simulink model "Blocks461_S20"  (R2017b)
settings: Solver=ode45  StartTime=0.  StopTime=20  MaxStep=0.01  RelTol=1e-6  AbsTol=1e-6  EnableMultiTasking=on
settings Model: ExtModeTrigMode=oneshot  ExtModeArmWhenConnect=off  Creator=LEVIENKL  LastModifiedBy=carlislt
settings DataIOCC: SaveFormat=Array  SignalLoggingSaveFormat=ModelDataLogs  SaveOutput=off  SaveTime=off  SignalLoggingName=sigsOut
settings OptimizationCC: BlockReduction=off  BooleanDataType=off  ExpressionDepthLimit=2147483647  InitFltsAndDblsToZero=on  LifeSpan=inf
settings DebuggingCC: SaveWithParameterizedLinksMsg=none  UnderspecifiedInitializationDetection=Classic  MergeDetectMultiDrivingBlocksExec=none  SignalResolutionControl=TryResolveAllWithWarning  MultiTaskDSMMsg=warning  MultiTaskCondExecSysMsg=none  FcnCallInpInsideContextMsg=warning  AllowSymbolicDim=off  StateNameClashWarn=warning  SFUnexpectedBacktrackingDiag=warning  SFNoUnconditionalDefaultTransitionDiag=warning  SFExecutionAtInitializationDiag=none
settings HardwareCC: ProdBitPerPointer=32  ProdBitPerSizeT=32  ProdBitPerPtrDiffT=32  ProdLargestAtomicFloat=None  ProdIntDivRoundTo=Undefined  ProdEndianess=Unspecified  ProdWordSize=32  ProdHWDeviceType=32-bit Generic  TargetUnknown=on
settings ModelReferenceCC: PropagateSignalLabelsOutOfModel=off
settings CodeAppCC: StateflowObjectComments=on
settings GRTTargetCC: TargetFcnLib=ansi_tfl_tmw.mat  TargetLangStandard=C89/C90 (ANSI)  GeneratePreprocessorConditionals=Disable all  CombineOutputUpdateFcns=off  GRTInterface=on
settings ConfigComp: CovMetricSettings=dw  CovHtmlReporting=on  CovSaveCumulativeToWorkspaceVar=on  CovSaveSingleToWorkspaceVar=on  CovExternalEMLEnable=off  CovSFcnEnable=off

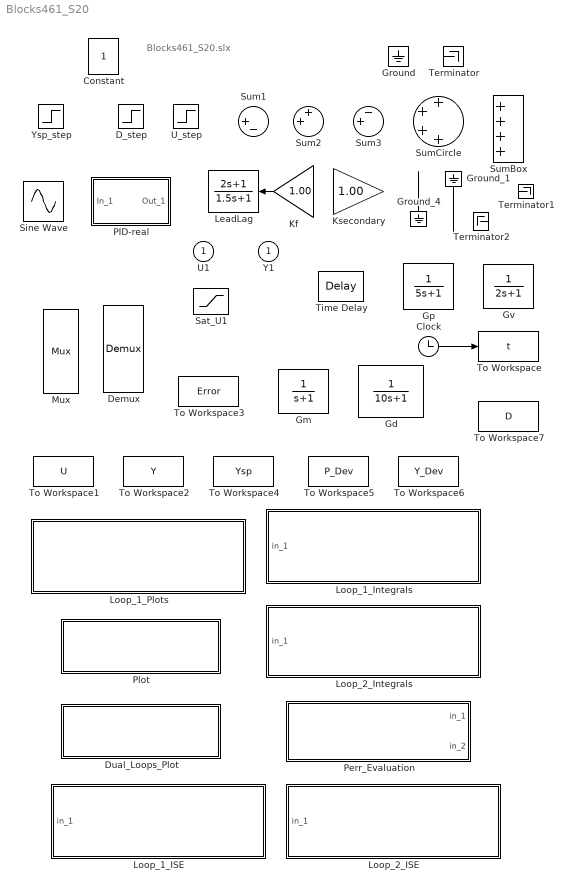
== system Blocks461_S20 ==
  note: Blocks461_S20.slx
  U1 : Inport
  Clock : Clock
  Constant : Constant
  D_step : Step  Time=0  After=0  SampleTime=0
      settings: AttributesFormatString=%<Before> to %<After>\nat %<Time>
  Demux : Demux  Outputs=2
  Dual_Loops_Plot : Subsystem  mask(Daul Y,P Plots 2 Loops){}
      settings: OpenFcn=DualYP
      mask Help: This block two loops Y and P.
      mask Display: disp('After Simulation:\n Double Click for Plots\n (uses DualYP.m)')
  Gd : TransferFcn  Denominator=[10 1]
  Gm : TransferFcn  Denominator=[1 1]
  "Gp " : TransferFcn  Denominator=[5 1]
  Ground : Ground
  Ground_1 : Ground
  Ground_4 : Ground
  Gv : TransferFcn  Denominator=[2 1]
  Kf : Gain  Gain=1.00  SaturateOnIntegerOverflow=on  OutDataTypeStr=Inherit: Same as input  ParamDataTypeStr=Inherit: Same as input
  Ksecondary : Gain  Gain=1.00  SaturateOnIntegerOverflow=on  OutDataTypeStr=Inherit: Same as input  ParamDataTypeStr=Inherit: Same as input
  LeadLag : TransferFcn  Numerator=[2, 1]  Denominator=[1.5, 1]
  Loop_1_ISE : Subsystem  mask(Integral Squarred Evaluation - Loop 1){}
      settings: OpenFcn=ISE1
      mask Help: This block calculates and plots loop #1 ISE.
      mask Display: disp('After Loop 1 Simulation:\n Double Click for ISE evaluation\n (uses ISE1.p)')
  Loop_1_Integrals : Subsystem  mask(Integral Error (3) Evaluations){}
      settings: OpenFcn=I3errs1
      mask Help: This block calculates loop #1 IAE, ISE and ITAE.
      mask Display: disp('After Loop 1 Simulation:\n Double Click for IAE, ISE & ITAE\n (uses I3errs1.p)')
  Loop_1_Plots : Subsystem  mask(Y,U,E Plots - Loop 1){}
      settings: OpenFcn=YPEplots
      mask Help: This block loop #1 Y,U,Error in 3x1 Figure Window.
      mask Display: disp('After Loop 1 Simulation:\n Double Click for Y, P, Error Plots\n (uses YPEplots.p)')
  Loop_2_ISE : Subsystem  mask(Integral Squarred Evaluation - Loop 2){}
      settings: OpenFcn=ISE2
      mask Help: This block calculates and plots loop #2 ISE.
      mask Display: disp('After Loop 2 Simulation:\n Double Click for ISE evaluation\n (uses ISE2.p)')
  Loop_2_Integrals : Subsystem  mask(3 Error evaluations){}
      settings: OpenFcn=I3errs2
      mask Help: This block calculates the IAE, the ISE and the ITAE.
      mask Display: disp('After Loop 2 Simulation:\n Double Click for IAE, ISE & ITAE\n (uses I3errs2.p)')
  Mux : Mux  Inputs=2
  PID-real : Subsystem  mask(PID(with alpha) Controller for ChE 461){Kc=1.00, tauIi=0, tauD=0, alpha=0.05}
      mask prompts: Kc "Controller gain:"; tauIi "Inv of Integral time constant (careful - this is I action ! ) :"; tauD "Derivative time constant:"; alpha "Alpha value (small)::"
      mask help:
      | Enter expressions for controller gain,
      | inverse of integral time constant
      | and derivative time constant and alpha.
      settings: AttributesFormatString=Kc = %<Kc>\n1/TauI = %<tauIi>\nTauD = %<tauD>
      mask Help: This block implements a PID controller where parameters are entered for the Controller Gain, inverse of Integral time constant and Derivative time constant.  Alpha here is equal to 0.01.   Unmask this block to see how it works. The derivative term is implemented using a true derivative block.
      mask Display: disp('PIDalpha')
  Perr_Evaluation : Subsystem  mask(Error evaluation){}
      settings: OpenFcn=Perror
      mask Help: This block calculates the average of the sum of ITAE and ISE for both outputs.
      mask Display: disp('After Project Simulation:\n Double Click for Project Error\n (uses Perror.p)')
  Plot : Subsystem  mask(Y,U,E Plots - Loop 1){}
      settings: OpenFcn=MyPlot
      mask Help: This block loop #1 Y,U,Error in 3x1 Figure Window.
      mask Display: disp('After Simulation:\n Double Click for Plots\n (uses MyPlot.m)')
  Sat_U1 : Saturate  UpperLimit=50  LowerLimit=-50  ZeroCross=off
      settings: AttributesFormatString=%<UpperLimit>\n%<LowerLimit>
  Sine Wave : Sin  SampleTime=0
      settings: AttributesFormatString=|
      | Amp = %<Amplitude>
      | Freq = %<Frequency> rad/t
  Sum1 : Sum  Inputs=|+-  SaturateOnIntegerOverflow=on  InputSameDT=on  OutDataTypeStr=Inherit: Same as first input
  Sum2 : Sum  Inputs=++|  SaturateOnIntegerOverflow=on  InputSameDT=on  OutDataTypeStr=Inherit: Same as first input
  Sum3 : Sum  Inputs=-+|  SaturateOnIntegerOverflow=on  InputSameDT=on  OutDataTypeStr=Inherit: Same as first input
  SumBox : Sum  Inputs=++++
  SumCircle : Sum  Inputs=++++
  Terminator : Terminator
  Terminator1 : Terminator
  Terminator2 : Terminator
  Time Delay : TransportDelay  DelayTime=0.5
      settings: AttributesFormatString=Delay=%<DelayTime>
  To Workspace : ToWorkspace  VariableName=t  SampleTime=-1
  To Workspace1 : ToWorkspace  VariableName=U  SampleTime=-1
  To Workspace2 : ToWorkspace  VariableName=Y  SampleTime=-1
  To Workspace3 : ToWorkspace  VariableName=Error  SampleTime=-1
  To Workspace4 : ToWorkspace  VariableName=Ysp  SampleTime=-1
  To Workspace5 : ToWorkspace  VariableName=P_Dev  SampleTime=-1
  To Workspace6 : ToWorkspace  VariableName=Y_Dev  SampleTime=-1
  To Workspace7 : ToWorkspace  VariableName=D  SampleTime=-1
  U_step : Step  Time=0  After=0  SampleTime=0
      settings: AttributesFormatString=%<Before> to %<After>\nat %<Time>
  Ysp_step : Step  Time=0  After=0  SampleTime=0
      settings: AttributesFormatString=%<Before> to %<After>\nat %<Time>
  Y1 : Outport
  wires:
  Ground_4/1 -> ?
  Ground_1/1 -> ?
  ? -> Terminator1/1
  ? -> Terminator2/1
  Clock/1 -> To Workspace/1
  Kf/1 -> LeadLag/1

== system Blocks461_S20/Dual_Loops_Plot ==

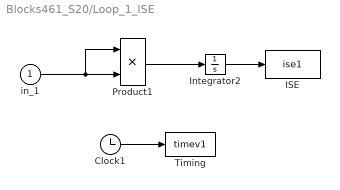
== system Blocks461_S20/Loop_1_ISE ==
  in_1 : Inport
  Clock1 : Clock
  ISE : ToWorkspace  VariableName=ise1
      settings: MaxDataPoints=20000
  Integrator2 : Integrator
  Product1 : Product  SaturateOnIntegerOverflow=on  RndMeth=Zero  InputSameDT=on  OutDataTypeStr=Inherit: Same as first input
  Timing : ToWorkspace  VariableName=timev1
      settings: MaxDataPoints=20000
  wires:
  Product1/1 -> Integrator2/1
  Clock1/1 -> Timing/1
  Integrator2/1 -> ISE/1
  in_1/1 -> Product1/1, Product1/2

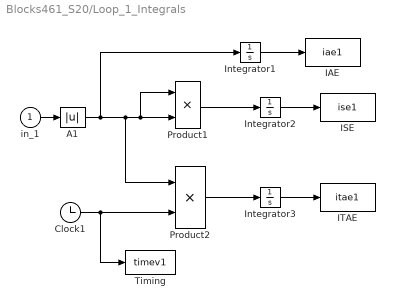
== system Blocks461_S20/Loop_1_Integrals ==
  in_1 : Inport
  A1 : Abs  ZeroCross=off  SaturateOnIntegerOverflow=on
  Clock1 : Clock
  IAE : ToWorkspace  VariableName=iae1
      settings: MaxDataPoints=20000
  ISE : ToWorkspace  VariableName=ise1
      settings: MaxDataPoints=20000
  ITAE : ToWorkspace  VariableName=itae1
      settings: MaxDataPoints=20000
  Integrator1 : Integrator
  Integrator2 : Integrator
  Integrator3 : Integrator
  Product1 : Product  SaturateOnIntegerOverflow=on  RndMeth=Zero  InputSameDT=on  OutDataTypeStr=Inherit: Same as first input
  Product2 : Product  SaturateOnIntegerOverflow=on  RndMeth=Zero  InputSameDT=on  OutDataTypeStr=Inherit: Same as first input
  Timing : ToWorkspace  VariableName=timev1
      settings: MaxDataPoints=20000
  wires:
  Integrator1/1 -> IAE/1
  Product1/1 -> Integrator2/1
  Clock1/1 -> Timing/1, Product2/2
  Integrator3/1 -> ITAE/1
  Integrator2/1 -> ISE/1
  Product2/1 -> Integrator3/1
  A1/1 -> Integrator1/1, Product2/1, Product1/1, Product1/2
  in_1/1 -> A1/1

== system Blocks461_S20/Loop_1_Plots ==

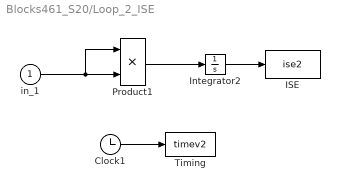
== system Blocks461_S20/Loop_2_ISE ==
  in_1 : Inport
  Clock1 : Clock
  ISE : ToWorkspace  VariableName=ise2
      settings: MaxDataPoints=20000
  Integrator2 : Integrator
  Product1 : Product  SaturateOnIntegerOverflow=on  RndMeth=Zero  InputSameDT=on  OutDataTypeStr=Inherit: Same as first input
  Timing : ToWorkspace  VariableName=timev2
      settings: MaxDataPoints=20000
  wires:
  Product1/1 -> Integrator2/1
  Clock1/1 -> Timing/1
  Integrator2/1 -> ISE/1
  in_1/1 -> Product1/1, Product1/2

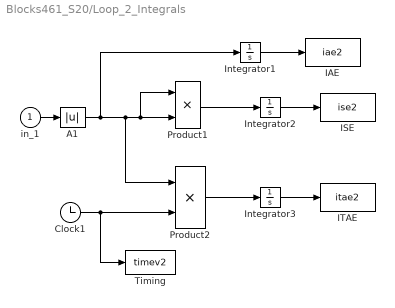
== system Blocks461_S20/Loop_2_Integrals ==
  in_1 : Inport
  A1 : Abs  ZeroCross=off  SaturateOnIntegerOverflow=on
  Clock1 : Clock
  IAE : ToWorkspace  VariableName=iae2
      settings: MaxDataPoints=20000
  ISE : ToWorkspace  VariableName=ise2
      settings: MaxDataPoints=20000
  ITAE : ToWorkspace  VariableName=itae2
      settings: MaxDataPoints=20000
  Integrator1 : Integrator
  Integrator2 : Integrator
  Integrator3 : Integrator
  Product1 : Product  SaturateOnIntegerOverflow=on  RndMeth=Zero  InputSameDT=on  OutDataTypeStr=Inherit: Same as first input
  Product2 : Product  SaturateOnIntegerOverflow=on  RndMeth=Zero  InputSameDT=on  OutDataTypeStr=Inherit: Same as first input
  Timing : ToWorkspace  VariableName=timev2
      settings: MaxDataPoints=20000
  wires:
  Integrator1/1 -> IAE/1
  Product1/1 -> Integrator2/1
  Clock1/1 -> Timing/1, Product2/2
  Integrator3/1 -> ITAE/1
  Integrator2/1 -> ISE/1
  Product2/1 -> Integrator3/1
  A1/1 -> Integrator1/1, Product2/1, Product1/1, Product1/2
  in_1/1 -> A1/1

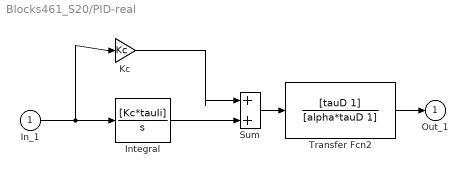
== system Blocks461_S20/PID-real ==
  In_1 : Inport
  Integral : TransferFcn  Numerator=[Kc*tauIi]  Denominator=[1 0]
  Kc : Gain  Gain=Kc  SaturateOnIntegerOverflow=on  OutDataTypeStr=Inherit: Same as input  ParamDataTypeStr=Inherit: Same as input
  Sum : Sum  SaturateOnIntegerOverflow=on  InputSameDT=on  OutDataTypeStr=Inherit: Same as first input
  Transfer Fcn2 : TransferFcn  Numerator=[tauD 1]  Denominator=[alpha*tauD 1]
  Out_1 : Outport
  wires:
  Kc/1 -> Sum/1
  Integral/1 -> Sum/2
  In_1/1 -> Kc/1, Integral/1
  Sum/1 -> Transfer Fcn2/1
  Transfer Fcn2/1 -> Out_1/1

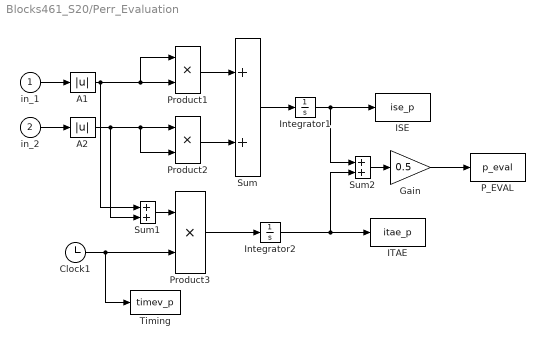
== system Blocks461_S20/Perr_Evaluation ==
  in_1 : Inport
  in_2 : Inport  Port=2
  A1 : Abs  ZeroCross=off  SaturateOnIntegerOverflow=on
  A2 : Abs  ZeroCross=off  SaturateOnIntegerOverflow=on
  Clock1 : Clock
  Gain : Gain  Gain=0.5  SaturateOnIntegerOverflow=on  OutDataTypeStr=Inherit: Same as input  ParamDataTypeStr=Inherit: Same as input
  ISE : ToWorkspace  VariableName=ise_p
      settings: MaxDataPoints=20000
  ITAE : ToWorkspace  VariableName=itae_p
      settings: MaxDataPoints=20000
  Integrator1 : Integrator
  Integrator2 : Integrator
  P_EVAL : ToWorkspace  VariableName=p_eval
      settings: MaxDataPoints=20000
  Product1 : Product  SaturateOnIntegerOverflow=on  RndMeth=Zero  InputSameDT=on  OutDataTypeStr=Inherit: Same as first input
  Product2 : Product  SaturateOnIntegerOverflow=on  RndMeth=Zero  InputSameDT=on  OutDataTypeStr=Inherit: Same as first input
  Product3 : Product  SaturateOnIntegerOverflow=on  RndMeth=Zero  InputSameDT=on  OutDataTypeStr=Inherit: Same as first input
  Sum : Sum  SaturateOnIntegerOverflow=on  InputSameDT=on  OutDataTypeStr=Inherit: Same as first input
  Sum1 : Sum  SaturateOnIntegerOverflow=on  InputSameDT=on  OutDataTypeStr=Inherit: Same as first input
  Sum2 : Sum  SaturateOnIntegerOverflow=on  InputSameDT=on  OutDataTypeStr=Inherit: Same as first input
  Timing : ToWorkspace  VariableName=timev_p
      settings: MaxDataPoints=20000
  wires:
  in_2/1 -> A2/1
  in_1/1 -> A1/1
  Product1/1 -> Sum/1
  Product2/1 -> Sum/2
  Sum/1 -> Integrator1/1
  Sum1/1 -> Product3/1
  A1/1 -> Product1/1, Product1/2, Sum1/1
  A2/1 -> Product2/2, Product2/1, Sum1/2
  Product3/1 -> Integrator2/1
  Integrator1/1 -> Sum2/1, ISE/1
  Integrator2/1 -> Sum2/2, ITAE/1
  Sum2/1 -> Gain/1
  Gain/1 -> P_EVAL/1
  Clock1/1 -> Timing/1, Product3/2

== system Blocks461_S20/Plot ==
